simulink subsystem "Wipers_Algorithm"  (R2025b)
settings: Solver=VariableStepAuto  StartTime=0.0  StopTime=10.0  RelTol=1e-3
libraries: simulink x7
settings Model: Creator=Sai Krishna  LastModifiedBy=Sai Krishna

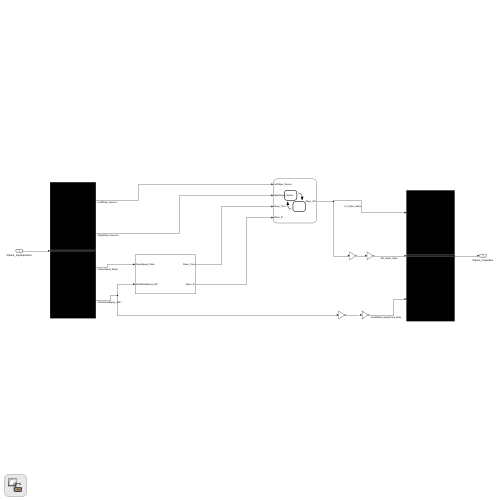
[thumbnail: Simulink's stored preview of the top-level diagram]
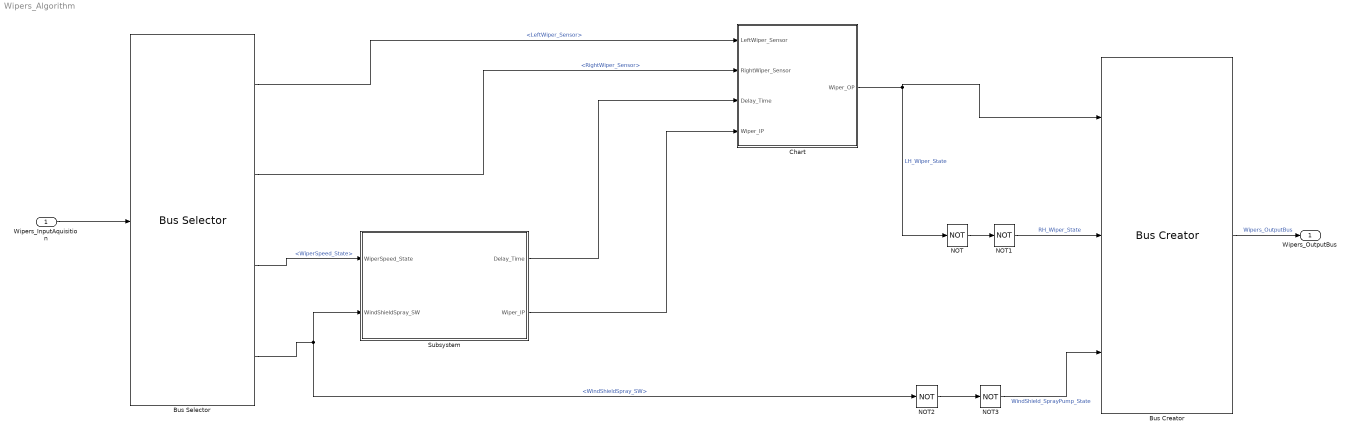
== system Wipers_Algorithm ==
  Wipers_InputAquisition : Inport  OutDataTypeStr=Bus: Wipers_InputBus
  Bus Creator : BusCreator  Inputs=3  OutDataTypeStr=Bus: Wipers_OutputBus
  Bus Selector : BusSelector  OutputSignals=LeftWiper_Sensor,RightWiper_Sensor,WiperSpeed_State,WindShieldSpray_SW
  Chart : Stateflow chart  TreatAsAtomicUnit=on
  NOT{,1..3} (4 alike) : Logic  Operator=NOT  IconShape=distinctive  AllPortsSameDT=off  OutDataTypeStr=boolean
  Subsystem : Subsystem
  Wipers_OutputBus : Outport  OutDataTypeStr=Bus: Wipers_OutputBus
  wires:
  Wipers_InputAquisition/1 -> Bus Selector/1
  Bus Creator/1 -> Wipers_OutputBus/1  "Wipers_OutputBus"
  Bus Selector/1 -> Chart/1(LeftWiper_Sensor)  "<LeftWiper_Sensor>"
  Bus Selector/2 -> Chart/2(RightWiper_Sensor)  "<RightWiper_Sensor>"
  Bus Selector/3 -> Subsystem/1(WiperSpeed_State)  "<WiperSpeed_State>"
  Subsystem/1(Delay_Time) -> Chart/3(Delay_Time)
  Subsystem/2(Wiper_IP) -> Chart/4(Wiper_IP)
  Bus Selector/4 -> Subsystem/2(WindShieldSpray_SW), NOT2/1  "<WindShieldSpray_SW>"
  Chart/1(Wiper_OP) -> NOT/1, Bus Creator/1  "LH_Wiper_State"
  NOT/1 -> NOT1/1
  NOT1/1 -> Bus Creator/2  "RH_Wiper_State"
  NOT2/1 -> NOT3/1
  NOT3/1 -> Bus Creator/3  "WindShield_SprayPump_State"

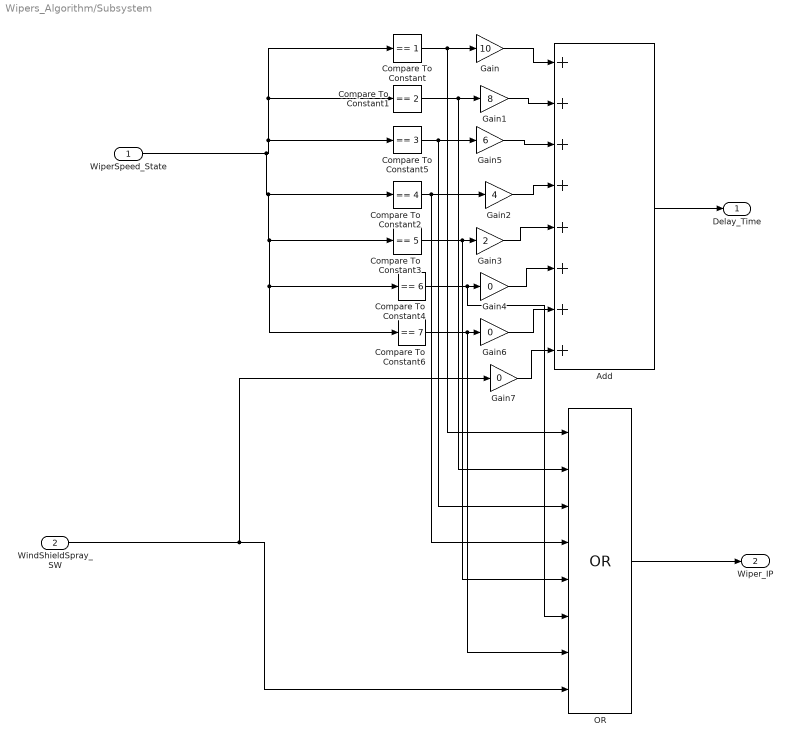
== system Wipers_Algorithm/Subsystem ==
  WiperSpeed_State : Inport
  WindShieldSpray_SW : Inport  Port=2
  Add : Sum  Inputs=++++++++
  Compare To Constant : simulink/Logic and Bit Operations/Compare To Constant  relop===  const=1  OutDataTypeStr=boolean
  Compare To Constant1 : simulink/Logic and Bit Operations/Compare To Constant  relop===  const=2  OutDataTypeStr=boolean
  Compare To Constant2 : simulink/Logic and Bit Operations/Compare To Constant  relop===  const=4  OutDataTypeStr=boolean
  Compare To Constant3 : simulink/Logic and Bit Operations/Compare To Constant  relop===  const=5  OutDataTypeStr=boolean
  Compare To Constant4 : simulink/Logic and Bit Operations/Compare To Constant  relop===  const=6  OutDataTypeStr=boolean
  Compare To Constant5 : simulink/Logic and Bit Operations/Compare To Constant  relop===  const=3  OutDataTypeStr=boolean
  Compare To Constant6 : simulink/Logic and Bit Operations/Compare To Constant  relop===  const=7  OutDataTypeStr=boolean
  Gain : Gain  Gain=10
  Gain1 : Gain  Gain=8
  Gain2 : Gain  Gain=4
  Gain3 : Gain  Gain=2
  Gain4 : Gain  Gain=0
  Gain5 : Gain  Gain=6
  Gain6 : Gain  Gain=0
  Gain7 : Gain  Gain=0
  OR : Logic  Operator=OR  Inputs=8  IconShape=distinctive  AllPortsSameDT=off  OutDataTypeStr=boolean
  Delay_Time : Outport
  Wiper_IP : Outport  Port=2
  wires:
  Gain7/1 -> Add/8
  WindShieldSpray_SW/1 -> OR/8, Gain7/1
  OR/1 -> Wiper_IP/1
  Add/1 -> Delay_Time/1
  Gain6/1 -> Add/7
  Gain4/1 -> Add/6
  Gain3/1 -> Add/5
  Gain2/1 -> Add/4
  Gain5/1 -> Add/3
  Gain1/1 -> Add/2
  Gain/1 -> Add/1
  WiperSpeed_State/1 -> Compare To Constant5/1, Compare To Constant1/1, Compare To Constant/1, Compare To Constant2/1, Compare To Constant3/1, Compare To Constant4/1, Compare To Constant6/1
  Compare To Constant6/1 -> Gain6/1, OR/7
  Compare To Constant5/1 -> Gain5/1, OR/3
  Compare To Constant4/1 -> Gain4/1, OR/6
  Compare To Constant3/1 -> Gain3/1, OR/5
  Compare To Constant2/1 -> Gain2/1, OR/4
  Compare To Constant1/1 -> Gain1/1, OR/2
  Compare To Constant/1 -> Gain/1, OR/1

== stateflow chart Wipers_Algorithm/Chart ==
  state OFF_
    Wiper_OP=false;
  state ON_
    Wiper_OP=true;
  state WAIT_
    Wiper_OP=false;
  (default) -> OFF_
  OFF_ -> ON_ : [LeftWiper_Sensor==true && RightWiper_Sensor==true && Wiper_IP==true]
  WAIT_ -> ON_ [order 1] : [after(Delay_Time, sec) && Wiper_IP==true]
  ON_ -> WAIT_ : [LeftWiper_Sensor==true && RightWiper_Sensor==true]
  WAIT_ -> OFF_ [order 2] : [Wiper_IP==false]
  data: LeftWiper_Sensor input; RightWiper_Sensor input; Delay_Time input; Wiper_IP input; Wiper_OP output
